simulink model "zad3_sim"  (R2022b)
settings: Solver=VariableStepAuto  StartTime=0.0  StopTime=9  RelTol=1e-3
values from neighbouring files (symbols this model uses):
  k1 = K(1)    [zad3.m]    (also in zadanie_dodatkowe.m)
  k2 = K(2)    [zad3.m]    (also in zadanie_dodatkowe.m)
  k3 = K(3)    [zad3.m]    (also in zadanie_dodatkowe.m)
settings Model: Creator=Mat  LastModifiedBy=Mat

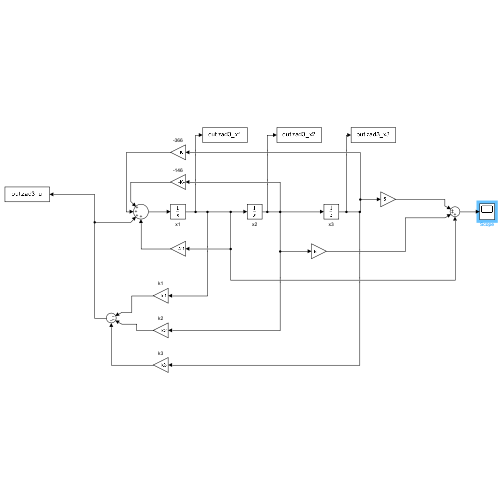
[thumbnail: Simulink's stored preview of the top-level diagram]
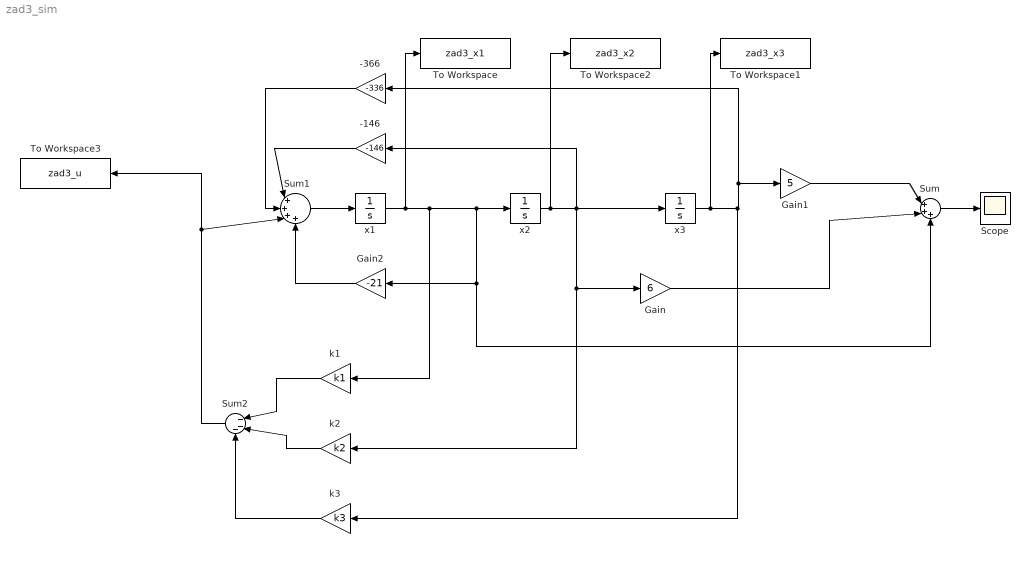
== system zad3_sim ==
  -146 : Gain  Gain=-146
  -366 : Gain  Gain=-336
  Gain : Gain  Gain=6
  Gain1 : Gain  Gain=5
  Gain2 : Gain  Gain=-21
  Scope : Scope
  Sum : Sum  Inputs=|+++
  Sum1 : Sum  Inputs=|++++
  Sum2 : Sum  Inputs=|---
  To Workspace : ToWorkspace  VariableName=zad3_x1  SaveFormat=Timeseries  SampleTime=-1
  To Workspace1 : ToWorkspace  VariableName=zad3_x3  SaveFormat=Timeseries  SampleTime=-1
  To Workspace2 : ToWorkspace  VariableName=zad3_x2  SaveFormat=Timeseries  SampleTime=-1
  To Workspace3 : ToWorkspace  VariableName=zad3_u  SaveFormat=Timeseries  SampleTime=-1
  k1 : Gain  Gain=k1
  k2 : Gain  Gain=k2
  k3 : Gain  Gain=k3
  x1 : Integrator  InitialCondition=-1
  x2 : Integrator  InitialCondition=-2
  x3 : Integrator  InitialCondition=-3
  wires:
  Sum1/1 -> x1/1
  Gain/1 -> Sum/2
  -366/1 -> Sum1/2
  Sum/1 -> Scope/1
  Gain1/1 -> Sum/1
  x2/1 -> To Workspace2/1, -146/1, x3/1, Gain/1, k2/1
  x1/1 -> To Workspace/1, k1/1, Gain2/1, Sum/3, x2/1
  -146/1 -> Sum1/1
  x3/1 -> To Workspace1/1, k3/1, Gain1/1, -366/1
  k1/1 -> Sum2/1
  k2/1 -> Sum2/2
  k3/1 -> Sum2/3
  Gain2/1 -> Sum1/4
  Sum2/1 -> To Workspace3/1, Sum1/3
